simulink model "Pilot_Assist"  (R2022b)
settings: configuration reference "CommonModelConfiguration" (kept outside this file)
undefined symbols (not defined in the file): cc_param_145, cc_param_311, LCFG_DSF_Timeout, LCFG_DSF_Timeout2, LCFG_PA_IntStsDelay, LCFG_VehicleBrand
settings Model: Creator=RPETE142  LastModifiedBy=OTHOMSO1
settings ConfigSetRef: SourceName=CommonModelConfiguration  SourceLocation=Base Workspace

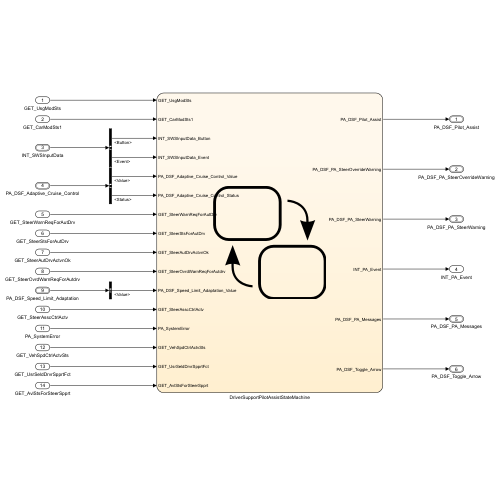
[thumbnail: Simulink's stored preview of the top-level diagram]
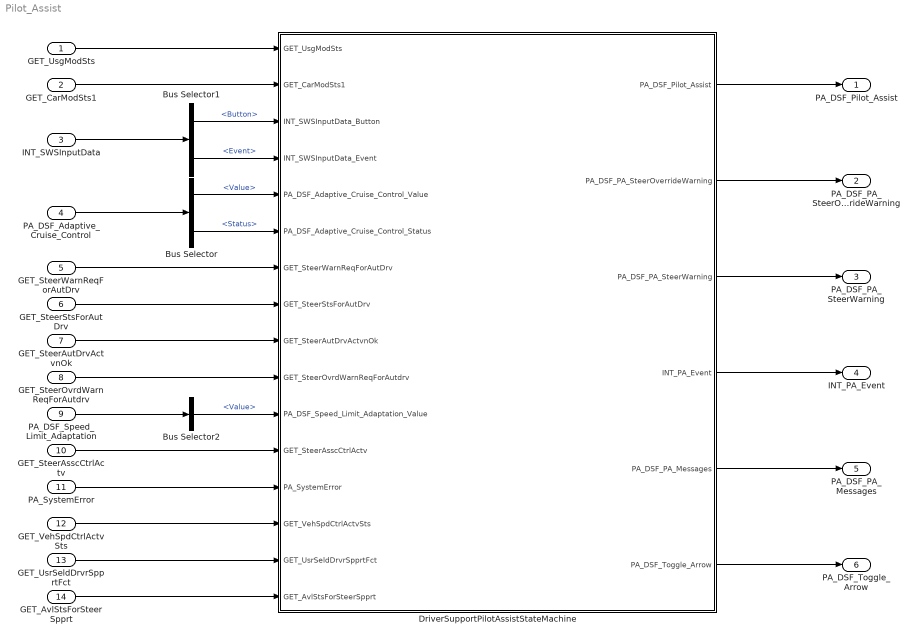
== system Pilot_Assist ==
  GET_UsgModSts : Inport  OutDataTypeStr=Enum: UsgModSts1
  GET_CarModSts1 : Inport  Port=2  OutDataTypeStr=Enum: CarModSts1
  INT_SWSInputData : Inport  Port=3  OutDataTypeStr=Bus: SWSInputData
  PA_DSF_Adaptive_Cruise_Control : Inport  Port=4  OutDataTypeStr=Bus: PA_DSF_ACC
  GET_SteerWarnReqForAutDrv : Inport  Port=5  OutDataTypeStr=Enum: SteerWarnReqForAutDrv1
  GET_SteerStsForAutDrv : Inport  Port=6  OutDataTypeStr=Enum: SteerStsForAutDrv3
  "GET_SteerAutDrvActvnOk " : Inport  Port=7  OutDataTypeStr=Enum: OnOff1
  GET_SteerOvrdWarnReqForAutdrv : Inport  Port=8  OutDataTypeStr=Enum: NoYesCrit1
  PA_DSF_Speed_Limit_Adaptation : Inport  Port=9  OutDataTypeStr=Bus: PA_DSF_SLA
  GET_SteerAsscCtrlActv : Inport  Port=10  OutDataTypeStr=Enum: OnOff1
  PA_SystemError : Inport  Port=11  OutDataTypeStr=boolean
  GET_VehSpdCtrlActvSts : Inport  Port=12  OutDataTypeStr=Enum: OnOff1
  GET_UsrSeldDrvrSpprtFct : Inport  Port=13  OutDataTypeStr=Enum: DrvrSpprtFct
  GET_AvlStsForSteerSpprt : Inport  Port=14  OutDataTypeStr=Enum: AvlStsForSteerSpprt1
  Bus Selector : BusSelector  OutputSignals=Value,Status
  Bus Selector1 : BusSelector  OutputSignals=Button,Event
  Bus Selector2 : BusSelector  OutputSignals=Value
  "DriverSupportPilotAssistStateMachine " : Stateflow chart  TreatAsAtomicUnit=on
  PA_DSF_Pilot_Assist : Outport  OutDataTypeStr=Bus: PA_DSF  VectorParamsAs1DForOutWhenUnconnected=off
  PA_DSF_PA_SteerOverrideWarning : Outport  Port=2  OutDataTypeStr=Bus: PA_StatusAndOffOnValue  VectorParamsAs1DForOutWhenUnconnected=off
  PA_DSF_PA_SteerWarning : Outport  Port=3  OutDataTypeStr=Bus: PA_DSF_SteerWarning  VectorParamsAs1DForOutWhenUnconnected=off
  INT_PA_Event : Outport  Port=4  OutDataTypeStr=Enum: E_DSF_Event  VectorParamsAs1DForOutWhenUnconnected=off
  PA_DSF_PA_Messages : Outport  Port=5  OutDataTypeStr=Bus: PA_DSF_Message  VectorParamsAs1DForOutWhenUnconnected=off  LockScale=on
  PA_DSF_Toggle_Arrow : Outport  Port=6  OutDataTypeStr=Bus: PA_StatusAndOffOnValue  VectorParamsAs1DForOutWhenUnconnected=off
  wires:
  GET_UsgModSts/1 -> "DriverSupportPilotAssistStateMachine "/1(GET_UsgModSts)
  GET_CarModSts1/1 -> "DriverSupportPilotAssistStateMachine "/2(GET_CarModSts1)
  Bus Selector/1 -> "DriverSupportPilotAssistStateMachine "/5(PA_DSF_Adaptive_Cruise_Control_Value)  "<Value>"
  PA_DSF_Adaptive_Cruise_Control/1 -> Bus Selector/1
  INT_SWSInputData/1 -> Bus Selector1/1
  Bus Selector1/2 -> "DriverSupportPilotAssistStateMachine "/4(INT_SWSInputData_Event)  "<Event>"
  Bus Selector1/1 -> "DriverSupportPilotAssistStateMachine "/3(INT_SWSInputData_Button)  "<Button>"
  PA_DSF_Speed_Limit_Adaptation/1 -> Bus Selector2/1
  PA_SystemError/1 -> "DriverSupportPilotAssistStateMachine "/13(PA_SystemError)
  GET_SteerStsForAutDrv/1 -> "DriverSupportPilotAssistStateMachine "/8(GET_SteerStsForAutDrv)
  GET_SteerWarnReqForAutDrv/1 -> "DriverSupportPilotAssistStateMachine "/7(GET_SteerWarnReqForAutDrv)
  "GET_SteerAutDrvActvnOk "/1 -> "DriverSupportPilotAssistStateMachine "/9(GET_SteerAutDrvActvnOk)
  GET_SteerOvrdWarnReqForAutdrv/1 -> "DriverSupportPilotAssistStateMachine "/10(GET_SteerOvrdWarnReqForAutdrv)
  "DriverSupportPilotAssistStateMachine "/1(PA_DSF_Pilot_Assist) -> PA_DSF_Pilot_Assist/1
  "DriverSupportPilotAssistStateMachine "/2(PA_DSF_PA_SteerOverrideWarning) -> PA_DSF_PA_SteerOverrideWarning/1
  "DriverSupportPilotAssistStateMachine "/3(PA_DSF_PA_SteerWarning) -> PA_DSF_PA_SteerWarning/1
  GET_SteerAsscCtrlActv/1 -> "DriverSupportPilotAssistStateMachine "/12(GET_SteerAsscCtrlActv)
  Bus Selector/2 -> "DriverSupportPilotAssistStateMachine "/6(PA_DSF_Adaptive_Cruise_Control_Status)  "<Status>"
  Bus Selector2/1 -> "DriverSupportPilotAssistStateMachine "/11(PA_DSF_Speed_Limit_Adaptation_Value)  "<Value>"
  "DriverSupportPilotAssistStateMachine "/4(INT_PA_Event) -> INT_PA_Event/1
  "DriverSupportPilotAssistStateMachine "/5(PA_DSF_PA_Messages) -> PA_DSF_PA_Messages/1
  GET_VehSpdCtrlActvSts/1 -> "DriverSupportPilotAssistStateMachine "/14(GET_VehSpdCtrlActvSts)
  GET_UsrSeldDrvrSpprtFct/1 -> "DriverSupportPilotAssistStateMachine "/15(GET_UsrSeldDrvrSpprtFct)
  GET_AvlStsForSteerSpprt/1 -> "DriverSupportPilotAssistStateMachine "/16(GET_AvlStsForSteerSpprt)
  "DriverSupportPilotAssistStateMachine "/6(PA_DSF_Toggle_Arrow) -> PA_DSF_Toggle_Arrow/1

== stateflow chart Pilot_Assist/DriverSupportPilotAssistStateMachine  ==
  state CARCONFIG_INVALID
    entry:
    PA_DSF_Pilot_Assist.Status = E_CommonStatus.NotPresent;
    PA_DSF_Pilot_Assist.Value = E_DSF_Value.DSF_Off;
    PA_DSF_PA_SteerOverrideWarning.Status = E_CommonStatus.NotPresent;
    PA_DSF_PA_SteerOverrideWarning.Value = E_OffOn.Off;
    PA_DSF_PA_SteerWarning.Status = E_CommonStatus.NotPresent;
    PA_DSF_PA_SteerWarning.Value = E_SteerWarning.SteerWarning_Off;
    INT_PA_Event = E_DSF_Event.Deactivation;
    PA_DSF_PA_Messages.Status = E_CommonStatus.NotPresent;
    PA_DSF_PA_Messages.Value = E_DSF_Messages.Messages_Off;
    PA_DSF_Toggle_Arrow.Status = E_CommonStatus.NotPresent;
    PA_DSF_Toggle_Arrow.Value = E_OffOn.Off;
  state SYSTEM_OK
    state isActive = activationCheck [function]
      (default) -> (junction 35)
      (junction 35) -> (junction 28) [order 1] : [GET_UsgModSts==UsgModSts1.UsgModSts1_UsgModDrvg &&...
          | GET_CarModSts1==CarModSts1.CarModSts1_CarModNorm &&...
          | PA_DSF_Adaptive_Cruise_Control_Status==E_CommonStatus.Available]
      (junction 35) -> (junction 29) [order 2] : {isActive = false;}
      (junction 28) -> (junction 30) : {isActive = true;}
      (junction 30) -> (junction 29)
      (junction 29) -> (junction 31)
    state NOT_ACTIVE
      entry:
      PA_DSF_Pilot_Assist.Status = E_CommonStatus.Disabled;
      PA_DSF_Pilot_Assist.Value = E_DSF_Value.DSF_Off;
      PA_DSF_PA_SteerOverrideWarning.Status = E_CommonStatus.Disabled;
      PA_DSF_PA_SteerOverrideWarning.Value = E_OffOn.Off;
      PA_DSF_PA_SteerWarning.Status = E_CommonStatus.Disabled;
      PA_DSF_PA_SteerWarning.Value = E_SteerWarning.SteerWarning_Off;
      INT_PA_Event = E_DSF_Event.Deactivation;
      PA_DSF_PA_Messages.Status = E_CommonStatus.Disabled;
      PA_DSF_PA_Messages.Value = E_DSF_Messages.Messages_Off;
      PA_DSF_Toggle_Arrow.Status = E_CommonStatus.Disabled;
      PA_DSF_Toggle_Arrow.Value = E_OffOn.Off;
    state ACTIVE
      entry:
      PA_DSF_PA_Messages.Status = E_CommonStatus.Available;
      PA_DSF_PA_Messages.Value = E_DSF_Messages.Messages_Off;
      PA_DSF_PA_SteerWarning.Status = E_CommonStatus.Available;
      PA_DSF_PA_SteerOverrideWarning.Status = E_CommonStatus.Available;
      PA_DSF_Pilot_Assist.Status = E_CommonStatus.Available;
      PA_DSF_Toggle_Arrow.Status = E_CommonStatus.Available;
      PA_DSF_Toggle_Arrow.Value = E_OffOn.Off;
      PA_Activated = true;
      state PILOT_ASSIST [parallel]
        settings: executionOrder=4
        state POLESTAR
          state HIDDEN
            entry:
            PA_DSF_Pilot_Assist.Value=E_DSF_Value.DSF_Off;
          state DISPLAYED
            state NOT_SELECTED
              entry:
              PA_DSF_Pilot_Assist.Value=E_DSF_Value.DSF_Not_Selected;
              INT_PA_Event = E_DSF_Event.Deactivation;
              isVisible = true;
            state SELECTED
              state ON
                entry:
                INT_PA_Event = E_DSF_Event.Activation;
                state ACTIVE
                  entry:
                  PA_DSF_Pilot_Assist.Value = E_DSF_Value.DSF_Active;
                state STANDBY
                  entry:
                  PA_DSF_Pilot_Assist.Value=E_DSF_Value.DSF_Standby;
                (default) -> (junction 2818)
                (junction 2818) -> (junction 2822) [order 2]
                (junction 2818) -> (junction 2823) [order 1] : [GET_SteerAsscCtrlActv  == OnOff1.OnOff1_On]
                (junction 2822) -> STANDBY
                (junction 2823) -> SYSTEM_OK.ACTIVE.PILOT_ASSIST.POLESTAR.DISPLAYED.SELECTED.ON.ACTIVE
                STANDBY -> SYSTEM_OK.ACTIVE.PILOT_ASSIST.POLESTAR.DISPLAYED.SELECTED.ON.ACTIVE : [GET_SteerAsscCtrlActv  == OnOff1.OnOff1_On]
                SYSTEM_OK.ACTIVE.PILOT_ASSIST.POLESTAR.DISPLAYED.SELECTED.ON.ACTIVE -> STANDBY : [GET_SteerAsscCtrlActv == OnOff1.OnOff1_Off]
              state OFF
                entry:
                PA_DSF_Pilot_Assist.Value=E_DSF_Value.DSF_Selected;
                INT_PA_Event = E_DSF_Event.Deactivation;
              (default) -> (junction 2801)
              (junction 2801) -> (junction 2804) [order 1] : [PA_DSF_Adaptive_Cruise_Control_Value == E_DSF_Value.DSF_Active || ...
                  | PA_DSF_Adaptive_Cruise_Control_Value == E_DSF_Value.DSF_StopMode]
              (junction 2801) -> OFF [order 2]
              (junction 2804) -> ON
              OFF -> ON [order 2] : [((hasChangedTo(PA_DSF_Adaptive_Cruise_Control_Value,E_DSF_Value.DSF_Active) || ...
                  | hasChangedTo(PA_DSF_Adaptive_Cruise_Control_Value,E_DSF_Value.DSF_StopMode)) && ...
                  | GET_SteerAutDrvActvnOk == OnOff1.OnOff1_On) ||...
                  | (after(LCFG_PA_IntStsDelay, sec) &&...
                  | (GET_SteerStsForAutDrv==SteerStsForAutDrv3.SteerStsForAutDrv3_Actv ||...
                  | GET_SteerStsForAutDrv==SteerStsForAutDrv3.SteerStsForAutDrv3_OvrdByDrvr))]
              ON -> OFF [order 1] : [PA_DSF_Adaptive_Cruise_Control_Value ~= E_DSF_Value.DSF_Active &&...
                  | PA_DSF_Adaptive_Cruise_Control_Value ~= E_DSF_Value.DSF_StopMode]
            (default) -> SYSTEM_OK.ACTIVE.PILOT_ASSIST.POLESTAR.DISPLAYED.NOT_SELECTED
            SYSTEM_OK.ACTIVE.PILOT_ASSIST.POLESTAR.DISPLAYED.NOT_SELECTED -> SYSTEM_OK.ACTIVE.PILOT_ASSIST.POLESTAR.DISPLAYED.SELECTED [order 1] : [INT_SWSInputData_Button == E_SWSButton.BtnL3Req &&...
                | hasChangedTo(INT_SWSInputData_Event, E_SWSEvent.Push) &&...
                | ((PA_DSF_Adaptive_Cruise_Control_Value ~= E_DSF_Value.DSF_Active &&...
                | PA_DSF_Adaptive_Cruise_Control_Value ~= E_DSF_Value.DSF_StopMode) ||...
                | GET_SteerAutDrvActvnOk == OnOff1.OnOff1_On)]
            SYSTEM_OK.ACTIVE.PILOT_ASSIST.POLESTAR.DISPLAYED.SELECTED -> SYSTEM_OK.ACTIVE.PILOT_ASSIST.POLESTAR.DISPLAYED.NOT_SELECTED : [INT_SWSInputData_Button == E_SWSButton.BtnL3Req &&...
                | hasChangedTo(INT_SWSInputData_Event, E_SWSEvent.Push)]
            SYSTEM_OK.ACTIVE.PILOT_ASSIST.POLESTAR.DISPLAYED.NOT_SELECTED -> ON [order 2] : [after(LCFG_PA_IntStsDelay, sec) &&...
                | (GET_SteerStsForAutDrv==SteerStsForAutDrv3.SteerStsForAutDrv3_Actv ||...
                | GET_SteerStsForAutDrv==SteerStsForAutDrv3.SteerStsForAutDrv3_OvrdByDrvr)]
            ON -> SYSTEM_OK.ACTIVE.PILOT_ASSIST.POLESTAR.DISPLAYED.NOT_SELECTED [order 2] : [(after(LCFG_PA_IntStsDelay, sec) &&...
                | GET_SteerStsForAutDrv~=SteerStsForAutDrv3.SteerStsForAutDrv3_Actv && ...
                | GET_SteerStsForAutDrv~=SteerStsForAutDrv3.SteerStsForAutDrv3_OvrdByDrvr)]
            OFF -> SYSTEM_OK.ACTIVE.PILOT_ASSIST.POLESTAR.DISPLAYED.NOT_SELECTED [order 1] : [(hasChangedTo(PA_DSF_Adaptive_Cruise_Control_Value,E_DSF_Value.DSF_Active) || ...
                | hasChangedTo(PA_DSF_Adaptive_Cruise_Control_Value,E_DSF_Value.DSF_StopMode)) && ...
                | GET_SteerAutDrvActvnOk == OnOff1.OnOff1_Off]
          (default) -> (junction 2539)
          (junction 2539) -> HIDDEN [order 1] : [isVisible == false && PA_DSF_Speed_Limit_Adaptation_Value == E_DSF_Value.DSF_Off]
          (junction 2539) -> DISPLAYED [order 2]
          HIDDEN -> DISPLAYED [order 2] : [PA_DSF_Adaptive_Cruise_Control_Value == E_DSF_Value.DSF_Active ||...
              | PA_DSF_Adaptive_Cruise_Control_Value == E_DSF_Value.DSF_StopMode ||...
              | PA_DSF_Speed_Limit_Adaptation_Value == E_DSF_Value.DSF_Selected]
          HIDDEN -> SYSTEM_OK.ACTIVE.PILOT_ASSIST.POLESTAR.DISPLAYED.SELECTED [order 1] : [INT_SWSInputData_Button == E_SWSButton.BtnL3Req &&...
              | hasChangedTo(INT_SWSInputData_Event, E_SWSEvent.Push)]
          HIDDEN -> ON [order 3] : [after(LCFG_PA_IntStsDelay, sec) &&...
              | (GET_SteerStsForAutDrv==SteerStsForAutDrv3.SteerStsForAutDrv3_Actv ||...
              | GET_SteerStsForAutDrv==SteerStsForAutDrv3.SteerStsForAutDrv3_OvrdByDrvr)]
        state PA_VOLVO
          %Toggle between PA and ACC with right button,
          %either in active or inactive (Argus3 only) mode
          state isA3 = Argus3 [function]
            (default) -> (junction 4176)
            (junction 4176) -> (junction 4177) [order 1] : [cc_param_311==3]
            (junction 4176) -> (junction 4178) [order 2] : {isA3 = false;}
            (junction 4177) -> (junction 4179) : {isA3 = true;}
            (junction 4179) -> (junction 4178)
            (junction 4178) -> (junction 4180)
          state isActive = ACC_active [function]
            (default) -> (junction 4163)
            (junction 4163) -> (junction 4164) [order 1] : [(PA_DSF_Adaptive_Cruise_Control_Value==E_DSF_Value.DSF_Active || ...
                | PA_DSF_Adaptive_Cruise_Control_Value==E_DSF_Value.DSF_StopMode)]
            (junction 4163) -> (junction 4165) [order 2] : {isActive = false;}
            (junction 4164) -> (junction 4166) : {isActive = true;}
            (junction 4166) -> (junction 4165)
            (junction 4165) -> (junction 4167)
          state SELECTED
            %Check if in active or inactive mode
            state ACC_ACTIVE
              %Send PA activation request and set PA active or
              %standby depending on steering assist availability
              entry:
              INT_PA_Event = E_DSF_Event.Activation;
              state PA_STANDBY
                entry:
                PA_DSF_Pilot_Assist.Value = E_DSF_Value.DSF_Standby;
              state PA_ACTIVE
                entry:
                PA_DSF_Pilot_Assist.Value = E_DSF_Value.DSF_Active;
              (default) -> (junction 4134)
              (junction 4134) -> PA_ACTIVE [order 1] : %Pilot Assist supports steering, normal PA symbol
                  | [GET_SteerAsscCtrlActv==OnOff1.OnOff1_On &&...
                  | PA_DSF_Adaptive_Cruise_Control_Value==E_DSF_Value.DSF_Active]
              (junction 4134) -> PA_STANDBY [order 2]
              PA_STANDBY -> PA_ACTIVE : %Pilot Assist supports steering, normal PA symbol
                  | [GET_SteerAsscCtrlActv==OnOff1.OnOff1_On &&...
                  | PA_DSF_Adaptive_Cruise_Control_Value==E_DSF_Value.DSF_Active]
              PA_ACTIVE -> PA_STANDBY : %Pilot Assist does not support steering, PA symbol with hands on wheel
                  | [GET_SteerAsscCtrlActv==OnOff1.OnOff1_Off ||...
                  | PA_DSF_Adaptive_Cruise_Control_Value==E_DSF_Value.DSF_StopMode]
            state ACC_NOT_ACTIVE
              %Set PA to selected, no activation
              entry:
              PA_DSF_Pilot_Assist.Value =...
              E_DSF_Value.DSF_Selected;
              INT_PA_Event = E_DSF_Event.NoReq;
            (default) -> (junction 4126)
            (junction 4126) -> ACC_ACTIVE [order 1] : %Display active PA symbol
                | [ACC_active]
            (junction 4126) -> ACC_NOT_ACTIVE [order 2]
            ACC_NOT_ACTIVE -> ACC_ACTIVE : %Display active PA symbol
                | [ACC_active]
            ACC_ACTIVE -> ACC_NOT_ACTIVE : %Display inactive PA symbol
                | [~ACC_active]
          state NOT_SELECTED
            %Set to not selected and send deactivation request if in active mode
            entry:
            PA_DSF_Pilot_Assist.Value = E_DSF_Value.DSF_Not_Selected;
            (default) -> (junction 4151)
            (junction 4151) -> (junction 4154) [order 1] : [ACC_active]
            (junction 4151) -> (junction 4150) [order 2] : {INT_PA_Event = E_DSF_Event.NoReq;}
            (junction 4154) -> (junction 4156) : {INT_PA_Event = E_DSF_Event.Deactivation;}
            (junction 4156) -> (junction 4150)
            (junction 4150) -> (junction 4159)
          (default) -> (junction 4122)
          (junction 4122) -> SYSTEM_OK.ACTIVE.PILOT_ASSIST.PA_VOLVO.SELECTED [order 1] : %Pilot Assist preselected by driver
              | [GET_VehSpdCtrlActvSts==OnOff1.OnOff1_On]
          (junction 4122) -> SYSTEM_OK.ACTIVE.PILOT_ASSIST.PA_VOLVO.NOT_SELECTED [order 2]
          SYSTEM_OK.ACTIVE.PILOT_ASSIST.PA_VOLVO.SELECTED -> SYSTEM_OK.ACTIVE.PILOT_ASSIST.PA_VOLVO.NOT_SELECTED : %Toggle Pilot Assist -> ACC (right button), in active mode only if not Argus3
              | [INT_SWSInputData_Button==E_SWSButton.BtnL3Req &&...
              | hasChangedTo(INT_SWSInputData_Event, E_SWSEvent.Push) &&...
              | (Argus3 || (~Argus3 && ACC_active))]
          SYSTEM_OK.ACTIVE.PILOT_ASSIST.PA_VOLVO.NOT_SELECTED -> SYSTEM_OK.ACTIVE.PILOT_ASSIST.PA_VOLVO.SELECTED : %Toggle ACC -> Pilot Assist (right button), in active mode only if not Argus3
              | [INT_SWSInputData_Button==E_SWSButton.BtnL3Req &&...
              | hasChangedTo(INT_SWSInputData_Event, E_SWSEvent.Push) &&...
              | (Argus3 || (~Argus3 && ACC_active))]
        (default) -> (junction 3374)
        (junction 3374) -> PA_VOLVO [order 2]
        (junction 3374) -> POLESTAR [order 1] : [LCFG_VehicleBrand==2]
      state MESSAGES [parallel]
        entry: PA_DSF_PA_Messages.Status = E_CommonStatus.Available;
        settings: executionOrder=1
        state retVal = paMessages [function]
          state retVal2 = paActivationReq [function]
            (default) -> (junction 4085)
            (junction 4085) -> (junction 4086) [order 1] : %Resume from standby with up button
                | [INT_SWSInputData_Button==E_SWSButton.BtnL5Req &&...
                | hasChangedTo(INT_SWSInputData_Event, E_SWSEvent.Push) &&...
                | GET_SteerAutDrvActvnOk==OnOff1.OnOff1_Off &&...
                | PA_DSF_Adaptive_Cruise_Control_Value==E_DSF_Value.DSF_Standby]
            (junction 4085) -> (junction 4087) [order 2]
            (junction 4086) -> (junction 4088)
            (junction 4087) -> (junction 4088) [order 1] : %Activate PA with middle button
                | [INT_SWSInputData_Button==E_SWSButton.BtnL1Req &&...
                | hasChangedTo(INT_SWSInputData_Event, E_SWSEvent.Push) &&...
                | GET_SteerAutDrvActvnOk==OnOff1.OnOff1_Off &&...
                | (PA_DSF_Adaptive_Cruise_Control_Value==E_DSF_Value.DSF_Standby ||...
                | PA_DSF_Adaptive_Cruise_Control_Value==E_DSF_Value.DSF_Selected)]
            (junction 4087) -> (junction 4089) [order 2]
            (junction 4088) -> (junction 4090)
            (junction 4089) -> (junction 4090) [order 1] : %Resume from stop mode with up button
                | [INT_SWSInputData_Button==E_SWSButton.BtnL5Req &&...
                | hasChangedTo(INT_SWSInputData_Event, E_SWSEvent.Push) &&...
                | PA_DSF_Adaptive_Cruise_Control_Value==E_DSF_Value.DSF_StopMode]
            (junction 4089) -> (junction 4091) [order 2]
            (junction 4090) -> (junction 4092)
            (junction 4091) -> (junction 4092) [order 1] : %Toggle from ACC to PA with right button
                | [INT_SWSInputData_Button==E_SWSButton.BtnL3Req &&...
                | hasChangedTo(INT_SWSInputData_Event, E_SWSEvent.Push) &&...
                | PA_DSF_Pilot_Assist.Value==E_DSF_Value.DSF_Not_Selected &&...
                | (PA_DSF_Adaptive_Cruise_Control_Value==E_DSF_Value.DSF_Active ||...
                | PA_DSF_Adaptive_Cruise_Control_Value==E_DSF_Value.DSF_StopMode)]
            (junction 4091) -> (junction 4093) [order 2] : {retVal2=false;}
            (junction 4092) -> (junction 4094) : {retVal2=true;}
            (junction 4094) -> (junction 4093)
            (junction 4093) -> (junction 4095)
          (default) -> (junction 4022)
          (junction 4022) -> (junction 4023) [order 1] : %Driver activation attempt
              | [paActivationReq()]
          (junction 4023) -> (junction 4024) [order 1] : [GET_AvlStsForSteerSpprt==AvlStsForSteerSpprt1.AvlStsForSteerSpprt_SteerUnavlTrailerAttached]
              | {PA_DSF_PA_Messages.Value = E_DSF_Messages.Messages_UnavailableTrailer;}
          (junction 4022) -> (junction 4031) [order 2]
          (junction 4023) -> (junction 4025) [order 2]
          (junction 4024) -> (junction 4026)
          (junction 4025) -> (junction 4026) [order 1] : [GET_AvlStsForSteerSpprt==AvlStsForSteerSpprt1.AvlStsForSteerSpprt_SteerUnavlRestOfDrive]
              | {PA_DSF_PA_Messages.Value = E_DSF_Messages.Messages_UnavailableWarningIgnored;}
          (junction 4025) -> (junction 4027) [order 2]
          (junction 4026) -> (junction 4028)
          (junction 4027) -> (junction 4028) [order 1] : [GET_AvlStsForSteerSpprt==AvlStsForSteerSpprt1.AvlStsForSteerSpprt_SteerUnavlDriverMontrUnavail]
              | {PA_DSF_PA_Messages.Value = E_DSF_Messages.Messages_UnavailableDriverMonitoring;}
          (junction 4027) -> (junction 4029) [order 2]
          (junction 4028) -> (junction 4030)
          (junction 4029) -> (junction 4030) [order 1] : [GET_AvlStsForSteerSpprt==AvlStsForSteerSpprt1.AvlStsForSteerSpprt_SteerUnavlSpdTooHigh]
              | {PA_DSF_PA_Messages.Value = E_DSF_Messages.Messages_UnavailableHighSpeed;}
          (junction 4029) -> (junction 4032) [order 2]
          (junction 4030) -> (junction 4033)
          (junction 4032) -> (junction 4031) [order 2]
          (junction 4032) -> (junction 4033) [order 1] : [GET_AvlStsForSteerSpprt==AvlStsForSteerSpprt1.AvlStsForSteerSpprt_SteerUnavlRoadEstNotPsbl]
              | {PA_DSF_PA_Messages.Value = E_DSF_Messages.Messages_UnavailableNoLanes;}
          (junction 4031) -> (junction 4188)
          (junction 4033) -> (junction 4036)
          (junction 4188) -> (junction 4112) [order 1] : %Steer assist has been cancelled
              | [hasChangedTo(GET_SteerAsscCtrlActv, OnOff1.OnOff1_Off)]
          (junction 4112) -> (junction 4036) [order 1] : [GET_AvlStsForSteerSpprt==AvlStsForSteerSpprt1.AvlStsForSteerSpprt_SteerUnavlRestOfDrive]
              | {PA_DSF_PA_Messages.Value = E_DSF_Messages.Messages_UnavailableWarningIgnored;}
          (junction 4188) -> (junction 4195) [order 2]
          (junction 4112) -> (junction 4114) [order 2]
          (junction 4036) -> (junction 4038)
          (junction 4114) -> (junction 4038) [order 1] : [GET_AvlStsForSteerSpprt==AvlStsForSteerSpprt1.AvlStsForSteerSpprt_SteerUnavlDriverMontrUnavail]
              | {PA_DSF_PA_Messages.Value = E_DSF_Messages.Messages_UnavailableDriverMonitoring;}
          (junction 4114) -> (junction 4115) [order 2]
          (junction 4038) -> (junction 4040)
          (junction 4115) -> (junction 4040) [order 1] : [GET_AvlStsForSteerSpprt==AvlStsForSteerSpprt1.AvlStsForSteerSpprt_SteerUnavlSpdTooHigh]
              | {PA_DSF_PA_Messages.Value = E_DSF_Messages.Messages_UnavailableHighSpeed;}
          (junction 4115) -> (junction 4116) [order 2]
          (junction 4040) -> (junction 4043)
          (junction 4116) -> (junction 4195) [order 2]
          (junction 4116) -> (junction 4043) [order 1] : [GET_AvlStsForSteerSpprt==AvlStsForSteerSpprt1.AvlStsForSteerSpprt_SteerUnavlRoadEstNotPsbl]
              | {PA_DSF_PA_Messages.Value = E_DSF_Messages.Messages_UnavailableNoLanes;}
          (junction 4195) -> (junction 4046) : {retVal = false;}
          (junction 4043) -> (junction 4045) : {retVal = true;}
          (junction 4045) -> (junction 4046)
          (junction 4046) -> (junction 4193)
        state HIDE_MESSAGES
          entry: PA_DSF_PA_Messages.Value =...
          E_DSF_Messages.Messages_Off;
        state SHOW_MESSAGES
        (default) -> HIDE_MESSAGES
        HIDE_MESSAGES -> SHOW_MESSAGES : [paMessages()]
        SHOW_MESSAGES -> HIDE_MESSAGES [order 2] : %PA reactivated or message timeout
            | [(hasChangedTo(GET_SteerAsscCtrlActv, OnOff1.OnOff1_On) &&...
            | PA_DSF_Adaptive_Cruise_Control_Value==E_DSF_Value.DSF_Active) ||...
            | after(LCFG_DSF_Timeout, sec)]
        SHOW_MESSAGES -> SHOW_MESSAGES [order 1] : [paMessages()]
      state WARNING_SOW [parallel]
        settings: executionOrder=2
        state NO_WARNING
          entry:
          PA_DSF_PA_SteerOverrideWarning.Value = E_OffOn.Off;
          note: 
        state WARNING
          entry:
          PA_DSF_PA_SteerOverrideWarning.Value = E_OffOn.On;
        (default) -> NO_WARNING
        WARNING -> NO_WARNING : [GET_SteerOvrdWarnReqForAutdrv ~= NoYesCrit1.NoYesCrit1_Yes ]
        NO_WARNING -> WARNING : [GET_SteerOvrdWarnReqForAutdrv == NoYesCrit1.NoYesCrit1_Yes ]
      state TOGGLE_ARROW [parallel]
        settings: executionOrder=5
        state SHOW_ARROW
          entry:
          PA_DSF_Toggle_Arrow.Value = E_OffOn.On;
        state HIDE_ARROW
          entry:
          PA_DSF_Toggle_Arrow.Value = E_OffOn.Off;
          note: 
        (default) -> HIDE_ARROW
        HIDE_ARROW -> SHOW_ARROW : %PA activated, middle or right button pushed
            | [PA_Activated || (INT_SWSInputData_Button==E_SWSButton.BtnL1Req ||...
            | INT_SWSInputData_Button==E_SWSButton.BtnL3Req) &&...
            | hasChangedTo(INT_SWSInputData_Event, E_SWSEvent.Push)]
        SHOW_ARROW -> HIDE_ARROW : [after(LCFG_DSF_Timeout2, sec)]
            | {PA_Activated = false;}
      state WARNING_SW [parallel]
        settings: executionOrder=3
        note: 
        (default) -> (junction 3126)
        WARNING_SW -> (junction 3126)
        (junction 3126) -> (junction 3125) [order 1] : [GET_SteerWarnReqForAutDrv == SteerWarnReqForAutDrv1.SteerWarnReqForAutDrv1_DispWarnForDrvrSteerLe]
            | {PA_DSF_PA_SteerWarning.Value = E_SteerWarning.SteerWarning_Left;}
        (junction 3126) -> (junction 3124) [order 2]
        (junction 3125) -> (junction 3119)
        (junction 3124) -> (junction 3119) [order 1] : [GET_SteerWarnReqForAutDrv == SteerWarnReqForAutDrv1.SteerWarnReqForAutDrv1_DispWarnForDrvrSteerRi]
            | {PA_DSF_PA_SteerWarning.Value = E_SteerWarning.SteerWarning_Right;}
        (junction 3119) -> (junction 3123)
        (junction 3124) -> (junction 3120) [order 2]
        (junction 3120) -> (junction 3123) [order 1] : [GET_SteerWarnReqForAutDrv == SteerWarnReqForAutDrv1.SteerWarnReqForAutDrv1_DispGenWarn]
            | {PA_DSF_PA_SteerWarning.Value = E_SteerWarning.SteerWarning_General;}
        (junction 3120) -> (junction 3111) [order 2] : {PA_DSF_PA_SteerWarning.Value = E_SteerWarning.SteerWarning_Off;}
        (junction 3123) -> (junction 3108)
        (junction 3108) -> (junction 3111)
        (junction 3111) -> (junction 3112)
    (default) -> (junction 3019)
    (junction 3019) -> NOT_ACTIVE [order 2]
    (junction 3019) -> (junction 3020) [order 1] : [activationCheck()]
    NOT_ACTIVE -> SYSTEM_OK.ACTIVE : [activationCheck()]
    SYSTEM_OK.ACTIVE -> NOT_ACTIVE : [~activationCheck()]
    (junction 3020) -> SYSTEM_OK.ACTIVE
  state ERROR
    entry:
    PA_DSF_Pilot_Assist.Status = E_CommonStatus.SystemError;
    PA_DSF_PA_SteerOverrideWarning.Status = E_CommonStatus.SystemError;
    PA_DSF_PA_SteerOverrideWarning.Value = E_OffOn.Off;
    PA_DSF_PA_SteerWarning.Status = E_CommonStatus.SystemError;
    PA_DSF_PA_SteerWarning.Value = E_SteerWarning.SteerWarning_Off;
    INT_PA_Event = E_DSF_Event.Deactivation;
    PA_DSF_PA_Messages.Status = E_CommonStatus.SystemError;
    PA_DSF_Toggle_Arrow.Status = E_CommonStatus.SystemError;
    PA_DSF_Toggle_Arrow.Value = E_OffOn.Off;
    state retVal = paActivationReq [function]
      (default) -> (junction 3007)
      (junction 3007) -> (junction 3008) [order 1] : [INT_SWSInputData_Button==E_SWSButton.BtnL3Req &&...
          | hasChangedTo(INT_SWSInputData_Event, E_SWSEvent.Push) &&...
          | PA_DSF_Adaptive_Cruise_Control_Status==E_CommonStatus.Available ]
      (junction 3007) -> (junction 3009) [order 2] : {retVal=false;}
      (junction 3008) -> (junction 3010) : {retVal=true;}
      (junction 3010) -> (junction 3009)
      (junction 3009) -> (junction 3011)
    state CANCEL_WARNING
      entry:
      PA_DSF_PA_Messages.Value = E_DSF_Messages.Messages_CancelWarning;
      PA_DSF_Pilot_Assist.Value = E_DSF_Value.DSF_Off;
    state UNAVAILABLE
      entry:
      PA_DSF_PA_Messages.Value = E_DSF_Messages.Messages_Unavailable;
    state NO_MESSAGES
      entry:
      PA_DSF_PA_Messages.Value = E_DSF_Messages.Messages_Off;
      PA_DSF_Pilot_Assist.Value = E_DSF_Value.DSF_Off;
    (default) -> (junction 3000)
    (junction 3000) -> (junction 2999) [order 1] : [PA_DSF_Pilot_Assist.Value==E_DSF_Value.DSF_Active ||...
        | PA_DSF_Pilot_Assist.Value==E_DSF_Value.DSF_Standby]
    UNAVAILABLE -> UNAVAILABLE [order 2] : [paActivationReq()]
    (junction 3000) -> NO_MESSAGES [order 2]
    (junction 2999) -> CANCEL_WARNING
    CANCEL_WARNING -> UNAVAILABLE [order 2] : [paActivationReq()]
    CANCEL_WARNING -> NO_MESSAGES [order 1] : [after(LCFG_DSF_Timeout, sec)]
    UNAVAILABLE -> NO_MESSAGES [order 1] : [after(LCFG_DSF_Timeout, sec)]
    NO_MESSAGES -> UNAVAILABLE : [paActivationReq()]
  (default) -> (junction 284)
  (junction 284) -> CARCONFIG_INVALID [order 2]
  (junction 284) -> (junction 287) [order 1] : [cc_param_145 > 2]
      | {PA_DSF_Pilot_Assist.Value =...
      | E_DSF_Value.DSF_Off;}
  (junction 287) -> SYSTEM_OK [order 2]
  (junction 287) -> (junction 1920) [order 1] : [PA_SystemError==true ||...
      | INT_SWSInputData_Event==...
      | E_SWSEvent.ButtonStuck]
  SYSTEM_OK -> ERROR : [PA_SystemError==true ||...
      | INT_SWSInputData_Event==...
      | E_SWSEvent.ButtonStuck]
  ERROR -> SYSTEM_OK : [PA_SystemError==false &&...
      | INT_SWSInputData_Event~=...
      | E_SWSEvent.ButtonStuck]
  (junction 1920) -> ERROR
  data: isActive function_output; isA3 function_output; isActive function_output; retVal2 function_output; retVal function_output; retVal function_output; GET_UsgModSts input Enum: UsgModSts1; GET_CarModSts1 input Enum: CarModSts1; INT_SWSInputData_Button input Enum: E_SWSButton; INT_SWSInputData_Event input Enum: E_SWSEvent; LCFG_PA_IntStsDelay parameter double; PA_DSF_Pilot_Assist output Bus: PA_DSF =0; PA_DSF_Adaptive_Cruise_Control_Value input Enum: E_DSF_Value; PA_DSF_Adaptive_Cruise_Control_Status input Enum: E_CommonStatus; PA_DSF_PA_SteerOverrideWarning output Bus: PA_StatusAndOffOnValue =0; PA_DSF_PA_SteerWarning output Bus: PA_DSF_SteerWarning =0; GET_SteerWarnReqForAutDrv input Enum: SteerWarnReqForAutDrv1; GET_SteerStsForAutDrv input Enum: SteerStsForAutDrv3; GET_SteerAutDrvActvnOk input Enum: OnOff1; GET_SteerOvrdWarnReqForAutdrv input Enum: NoYesCrit1; PA_DSF_Speed_Limit_Adaptation_Value input Enum: E_DSF_Value; cc_param_145 parameter double; GET_SteerAsscCtrlActv input Enum: OnOff1; PA_SystemError input boolean; isVisible local boolean =false; INT_PA_Event output Enum: E_DSF_Event; LCFG_DSF_Timeout2 parameter; PA_DSF_PA_Messages output Bus: PA_DSF_Message; LCFG_DSF_Timeout parameter; LCFG_VehicleBrand parameter single; GET_VehSpdCtrlActvSts input Enum: OnOff1; GET_UsrSeldDrvrSpprtFct input Enum: DrvrSpprtFct; GET_AvlStsForSteerSpprt input Enum: AvlStsForSteerSpprt1; PA_DSF_Toggle_Arrow output Bus: PA_StatusAndOffOnValue; PA_Activated local boolean; cc_param_311 parameter double
